simulink subsystem "DetailedBatteryModel"  (R2023b)
settings: Solver=VariableStepAuto  StartTime=0.0  StopTime=10.0  RelTol=1e-3
undefined symbols (not defined in the file): PlntBattBalSwtchThresh, PlntBattBleedRes, PlntBattCondArea, PlntBattNumCellPar, ThrmBatt1, ThrmBatt2, ThrmBatt3, ThrmBatt4
libraries: fl_lib x580, nesl_utility_internal x386, batteryecm_lib x96, simulink x96
(part 7 of 7)

== system DetailedBatteryModel/BatteryPack_16Modules/Cell_Module_2/s15 ==
  Compare To Constant4 : simulink/Logic and Bit Operations/Compare To Constant  relop=<=  const=0.001  OutDataTypeStr=boolean
  PS-Simulink Converter10 : nesl_utility_internal/PS-Simulink Converter  PhysicalDomain=network_engine_domain  SubClassName=ps_output  LeftPortType=input  RightPortType=output  PseudoPeriodic=off  Frequencies=[]  VectorFormat=1-D array  Unit=1  AffineConversion=off
  Stop Simulation4 : Stop
  p : PMIOPort  Side=Left
  wires:
  PS-Simulink Converter10/1 -> Compare To Constant4/1
  Compare To Constant4/1 -> Stop Simulation4/1
  connections:
  PS-Simulink Converter10/LConn1 -- p/RConn1

== system DetailedBatteryModel/BatteryPack_16Modules/Cell_Module_2/s16 ==
  Compare To Constant5 : simulink/Logic and Bit Operations/Compare To Constant  relop=<=  const=0.001  OutDataTypeStr=boolean
  PS-Simulink Converter11 : nesl_utility_internal/PS-Simulink Converter  PhysicalDomain=network_engine_domain  SubClassName=ps_output  LeftPortType=input  RightPortType=output  PseudoPeriodic=off  Frequencies=[]  VectorFormat=1-D array  Unit=1  AffineConversion=off
  Stop Simulation5 : Stop
  p : PMIOPort  Side=Left
  wires:
  PS-Simulink Converter11/1 -> Compare To Constant5/1
  Compare To Constant5/1 -> Stop Simulation5/1
  connections:
  PS-Simulink Converter11/LConn1 -- p/RConn1

== system DetailedBatteryModel/BatteryPack_16Modules/Cell_Module_2/s17 ==
  Compare To Constant1 : simulink/Logic and Bit Operations/Compare To Constant  relop=<=  const=0.001  OutDataTypeStr=boolean
  PS-Simulink Converter7 : nesl_utility_internal/PS-Simulink Converter  PhysicalDomain=network_engine_domain  SubClassName=ps_output  LeftPortType=input  RightPortType=output  PseudoPeriodic=off  Frequencies=[]  VectorFormat=1-D array  Unit=1  AffineConversion=off
  Stop Simulation1 : Stop
  p : PMIOPort  Side=Left
  wires:
  PS-Simulink Converter7/1 -> Compare To Constant1/1
  Compare To Constant1/1 -> Stop Simulation1/1
  connections:
  PS-Simulink Converter7/LConn1 -- p/RConn1

== system DetailedBatteryModel/BatteryPack_16Modules/Cell_Module_2/s18 ==
  Compare To Constant2 : simulink/Logic and Bit Operations/Compare To Constant  relop=<=  const=0.001  OutDataTypeStr=boolean
  PS-Simulink Converter8 : nesl_utility_internal/PS-Simulink Converter  PhysicalDomain=network_engine_domain  SubClassName=ps_output  LeftPortType=input  RightPortType=output  PseudoPeriodic=off  Frequencies=[]  VectorFormat=1-D array  Unit=1  AffineConversion=off
  Stop Simulation2 : Stop
  p : PMIOPort  Side=Left
  wires:
  Compare To Constant2/1 -> Stop Simulation2/1
  PS-Simulink Converter8/1 -> Compare To Constant2/1
  connections:
  PS-Simulink Converter8/LConn1 -- p/RConn1

== system DetailedBatteryModel/BatteryPack_16Modules/Cell_Module_2/s19 ==
  Compare To Constant3 : simulink/Logic and Bit Operations/Compare To Constant  relop=<=  const=0.001  OutDataTypeStr=boolean
  PS-Simulink Converter9 : nesl_utility_internal/PS-Simulink Converter  PhysicalDomain=network_engine_domain  SubClassName=ps_output  LeftPortType=input  RightPortType=output  PseudoPeriodic=off  Frequencies=[]  VectorFormat=1-D array  Unit=1  AffineConversion=off
  Stop Simulation3 : Stop
  p : PMIOPort  Side=Left
  wires:
  PS-Simulink Converter9/1 -> Compare To Constant3/1
  Compare To Constant3/1 -> Stop Simulation3/1
  connections:
  PS-Simulink Converter9/LConn1 -- p/RConn1

== system DetailedBatteryModel/BatteryPack_16Modules/Cell_Module_2/s2 ==
  Compare To Constant3 : simulink/Logic and Bit Operations/Compare To Constant  relop=<=  const=0.001  OutDataTypeStr=boolean
  PS-Simulink Converter9 : nesl_utility_internal/PS-Simulink Converter  PhysicalDomain=network_engine_domain  SubClassName=ps_output  LeftPortType=input  RightPortType=output  PseudoPeriodic=off  Frequencies=[]  VectorFormat=1-D array  Unit=1  AffineConversion=off
  Stop Simulation3 : Stop
  p : PMIOPort  Side=Left
  wires:
  PS-Simulink Converter9/1 -> Compare To Constant3/1
  Compare To Constant3/1 -> Stop Simulation3/1
  connections:
  PS-Simulink Converter9/LConn1 -- p/RConn1

== system DetailedBatteryModel/BatteryPack_16Modules/Cell_Module_2/s20 ==
  Compare To Constant4 : simulink/Logic and Bit Operations/Compare To Constant  relop=<=  const=0.001  OutDataTypeStr=boolean
  PS-Simulink Converter10 : nesl_utility_internal/PS-Simulink Converter  PhysicalDomain=network_engine_domain  SubClassName=ps_output  LeftPortType=input  RightPortType=output  PseudoPeriodic=off  Frequencies=[]  VectorFormat=1-D array  Unit=1  AffineConversion=off
  Stop Simulation4 : Stop
  p : PMIOPort  Side=Left
  wires:
  PS-Simulink Converter10/1 -> Compare To Constant4/1
  Compare To Constant4/1 -> Stop Simulation4/1
  connections:
  PS-Simulink Converter10/LConn1 -- p/RConn1

== system DetailedBatteryModel/BatteryPack_16Modules/Cell_Module_2/s21 ==
  Compare To Constant5 : simulink/Logic and Bit Operations/Compare To Constant  relop=<=  const=0.001  OutDataTypeStr=boolean
  PS-Simulink Converter11 : nesl_utility_internal/PS-Simulink Converter  PhysicalDomain=network_engine_domain  SubClassName=ps_output  LeftPortType=input  RightPortType=output  PseudoPeriodic=off  Frequencies=[]  VectorFormat=1-D array  Unit=1  AffineConversion=off
  Stop Simulation5 : Stop
  p : PMIOPort  Side=Left
  wires:
  PS-Simulink Converter11/1 -> Compare To Constant5/1
  Compare To Constant5/1 -> Stop Simulation5/1
  connections:
  PS-Simulink Converter11/LConn1 -- p/RConn1

== system DetailedBatteryModel/BatteryPack_16Modules/Cell_Module_2/s22 ==
  Compare To Constant5 : simulink/Logic and Bit Operations/Compare To Constant  relop=<=  const=0.001  OutDataTypeStr=boolean
  PS-Simulink Converter11 : nesl_utility_internal/PS-Simulink Converter  PhysicalDomain=network_engine_domain  SubClassName=ps_output  LeftPortType=input  RightPortType=output  PseudoPeriodic=off  Frequencies=[]  VectorFormat=1-D array  Unit=1  AffineConversion=off
  Stop Simulation5 : Stop
  p : PMIOPort  Side=Left
  wires:
  Compare To Constant5/1 -> Stop Simulation5/1
  PS-Simulink Converter11/1 -> Compare To Constant5/1
  connections:
  PS-Simulink Converter11/LConn1 -- p/RConn1

== system DetailedBatteryModel/BatteryPack_16Modules/Cell_Module_2/s3 ==
  Compare To Constant4 : simulink/Logic and Bit Operations/Compare To Constant  relop=<=  const=0.001  OutDataTypeStr=boolean
  PS-Simulink Converter10 : nesl_utility_internal/PS-Simulink Converter  PhysicalDomain=network_engine_domain  SubClassName=ps_output  LeftPortType=input  RightPortType=output  PseudoPeriodic=off  Frequencies=[]  VectorFormat=1-D array  Unit=1  AffineConversion=off
  Stop Simulation4 : Stop
  p : PMIOPort  Side=Left
  wires:
  PS-Simulink Converter10/1 -> Compare To Constant4/1
  Compare To Constant4/1 -> Stop Simulation4/1
  connections:
  PS-Simulink Converter10/LConn1 -- p/RConn1

== system DetailedBatteryModel/BatteryPack_16Modules/Cell_Module_2/s4 ==
  Compare To Constant5 : simulink/Logic and Bit Operations/Compare To Constant  relop=<=  const=0.001  OutDataTypeStr=boolean
  PS-Simulink Converter11 : nesl_utility_internal/PS-Simulink Converter  PhysicalDomain=network_engine_domain  SubClassName=ps_output  LeftPortType=input  RightPortType=output  PseudoPeriodic=off  Frequencies=[]  VectorFormat=1-D array  Unit=1  AffineConversion=off
  Stop Simulation5 : Stop
  p : PMIOPort  Side=Left
  wires:
  PS-Simulink Converter11/1 -> Compare To Constant5/1
  Compare To Constant5/1 -> Stop Simulation5/1
  connections:
  PS-Simulink Converter11/LConn1 -- p/RConn1

== system DetailedBatteryModel/BatteryPack_16Modules/Cell_Module_2/s5 ==
  Compare To Constant1 : simulink/Logic and Bit Operations/Compare To Constant  relop=<=  const=0.001  OutDataTypeStr=boolean
  PS-Simulink Converter7 : nesl_utility_internal/PS-Simulink Converter  PhysicalDomain=network_engine_domain  SubClassName=ps_output  LeftPortType=input  RightPortType=output  PseudoPeriodic=off  Frequencies=[]  VectorFormat=1-D array  Unit=1  AffineConversion=off
  Stop Simulation1 : Stop
  p : PMIOPort  Side=Left
  wires:
  PS-Simulink Converter7/1 -> Compare To Constant1/1
  Compare To Constant1/1 -> Stop Simulation1/1
  connections:
  PS-Simulink Converter7/LConn1 -- p/RConn1

== system DetailedBatteryModel/BatteryPack_16Modules/Cell_Module_2/s6 ==
  Compare To Constant2 : simulink/Logic and Bit Operations/Compare To Constant  relop=<=  const=0.001  OutDataTypeStr=boolean
  PS-Simulink Converter8 : nesl_utility_internal/PS-Simulink Converter  PhysicalDomain=network_engine_domain  SubClassName=ps_output  LeftPortType=input  RightPortType=output  PseudoPeriodic=off  Frequencies=[]  VectorFormat=1-D array  Unit=1  AffineConversion=off
  Stop Simulation2 : Stop
  p : PMIOPort  Side=Left
  wires:
  Compare To Constant2/1 -> Stop Simulation2/1
  PS-Simulink Converter8/1 -> Compare To Constant2/1
  connections:
  PS-Simulink Converter8/LConn1 -- p/RConn1

== system DetailedBatteryModel/BatteryPack_16Modules/Cell_Module_2/s7 ==
  Compare To Constant3 : simulink/Logic and Bit Operations/Compare To Constant  relop=<=  const=0.001  OutDataTypeStr=boolean
  PS-Simulink Converter9 : nesl_utility_internal/PS-Simulink Converter  PhysicalDomain=network_engine_domain  SubClassName=ps_output  LeftPortType=input  RightPortType=output  PseudoPeriodic=off  Frequencies=[]  VectorFormat=1-D array  Unit=1  AffineConversion=off
  Stop Simulation3 : Stop
  p : PMIOPort  Side=Left
  wires:
  PS-Simulink Converter9/1 -> Compare To Constant3/1
  Compare To Constant3/1 -> Stop Simulation3/1
  connections:
  PS-Simulink Converter9/LConn1 -- p/RConn1

== system DetailedBatteryModel/BatteryPack_16Modules/Cell_Module_2/s8 ==
  Compare To Constant4 : simulink/Logic and Bit Operations/Compare To Constant  relop=<=  const=0.001  OutDataTypeStr=boolean
  PS-Simulink Converter10 : nesl_utility_internal/PS-Simulink Converter  PhysicalDomain=network_engine_domain  SubClassName=ps_output  LeftPortType=input  RightPortType=output  PseudoPeriodic=off  Frequencies=[]  VectorFormat=1-D array  Unit=1  AffineConversion=off
  Stop Simulation4 : Stop
  p : PMIOPort  Side=Left
  wires:
  PS-Simulink Converter10/1 -> Compare To Constant4/1
  Compare To Constant4/1 -> Stop Simulation4/1
  connections:
  PS-Simulink Converter10/LConn1 -- p/RConn1

== system DetailedBatteryModel/BatteryPack_16Modules/Cell_Module_2/s9 ==
  Compare To Constant5 : simulink/Logic and Bit Operations/Compare To Constant  relop=<=  const=0.001  OutDataTypeStr=boolean
  PS-Simulink Converter11 : nesl_utility_internal/PS-Simulink Converter  PhysicalDomain=network_engine_domain  SubClassName=ps_output  LeftPortType=input  RightPortType=output  PseudoPeriodic=off  Frequencies=[]  VectorFormat=1-D array  Unit=1  AffineConversion=off
  Stop Simulation5 : Stop
  p : PMIOPort  Side=Left
  wires:
  PS-Simulink Converter11/1 -> Compare To Constant5/1
  Compare To Constant5/1 -> Stop Simulation5/1
  connections:
  PS-Simulink Converter11/LConn1 -- p/RConn1

== system DetailedBatteryModel/BatteryPack_16Modules/Cell_Module_3/Subsystem ==
  Compare To Constant : simulink/Logic and Bit Operations/Compare To Constant  relop=<=  const=0.001  OutDataTypeStr=boolean
  Data Type Conversion6 : DataTypeConversion  OutDataTypeStr=single  SaturateOnIntegerOverflow=off  RndMeth=Floor
  PS-Simulink Converter6 : nesl_utility_internal/PS-Simulink Converter  PhysicalDomain=network_engine_domain  SubClassName=ps_output  LeftPortType=input  RightPortType=output  PseudoPeriodic=off  Frequencies=[]  VectorFormat=1-D array  Unit=1  AffineConversion=off
  Stop Simulation : Stop
  P : PMIOPort  Side=Left
  soc : Outport
  wires:
  Data Type Conversion6/1 -> soc/1  "KnownSOC"
  PS-Simulink Converter6/1 -> Compare To Constant/1, Data Type Conversion6/1  "KnownSOC"
  Compare To Constant/1 -> Stop Simulation/1
  connections:
  P/RConn1 -- PS-Simulink Converter6/LConn1

== system DetailedBatteryModel/BatteryPack_16Modules/Cell_Module_3/s ==
  Compare To Constant1 : simulink/Logic and Bit Operations/Compare To Constant  relop=<=  const=0.001  OutDataTypeStr=boolean
  PS-Simulink Converter7 : nesl_utility_internal/PS-Simulink Converter  PhysicalDomain=network_engine_domain  SubClassName=ps_output  LeftPortType=input  RightPortType=output  PseudoPeriodic=off  Frequencies=[]  VectorFormat=1-D array  Unit=1  AffineConversion=off
  Stop Simulation1 : Stop
  p : PMIOPort  Side=Left
  wires:
  PS-Simulink Converter7/1 -> Compare To Constant1/1
  Compare To Constant1/1 -> Stop Simulation1/1
  connections:
  PS-Simulink Converter7/LConn1 -- p/RConn1

== system DetailedBatteryModel/BatteryPack_16Modules/Cell_Module_3/s1 ==
  Compare To Constant2 : simulink/Logic and Bit Operations/Compare To Constant  relop=<=  const=0.001  OutDataTypeStr=boolean
  PS-Simulink Converter8 : nesl_utility_internal/PS-Simulink Converter  PhysicalDomain=network_engine_domain  SubClassName=ps_output  LeftPortType=input  RightPortType=output  PseudoPeriodic=off  Frequencies=[]  VectorFormat=1-D array  Unit=1  AffineConversion=off
  Stop Simulation2 : Stop
  p : PMIOPort  Side=Left
  wires:
  Compare To Constant2/1 -> Stop Simulation2/1
  PS-Simulink Converter8/1 -> Compare To Constant2/1
  connections:
  PS-Simulink Converter8/LConn1 -- p/RConn1

== system DetailedBatteryModel/BatteryPack_16Modules/Cell_Module_3/s10 ==
  Compare To Constant5 : simulink/Logic and Bit Operations/Compare To Constant  relop=<=  const=0.001  OutDataTypeStr=boolean
  PS-Simulink Converter11 : nesl_utility_internal/PS-Simulink Converter  PhysicalDomain=network_engine_domain  SubClassName=ps_output  LeftPortType=input  RightPortType=output  PseudoPeriodic=off  Frequencies=[]  VectorFormat=1-D array  Unit=1  AffineConversion=off
  Stop Simulation5 : Stop
  p : PMIOPort  Side=Left
  wires:
  Compare To Constant5/1 -> Stop Simulation5/1
  PS-Simulink Converter11/1 -> Compare To Constant5/1
  connections:
  PS-Simulink Converter11/LConn1 -- p/RConn1

== system DetailedBatteryModel/BatteryPack_16Modules/Cell_Module_3/s11 ==
  Compare To Constant1 : simulink/Logic and Bit Operations/Compare To Constant  relop=<=  const=0.001  OutDataTypeStr=boolean
  PS-Simulink Converter7 : nesl_utility_internal/PS-Simulink Converter  PhysicalDomain=network_engine_domain  SubClassName=ps_output  LeftPortType=input  RightPortType=output  PseudoPeriodic=off  Frequencies=[]  VectorFormat=1-D array  Unit=1  AffineConversion=off
  Stop Simulation1 : Stop
  p : PMIOPort  Side=Left
  wires:
  PS-Simulink Converter7/1 -> Compare To Constant1/1
  Compare To Constant1/1 -> Stop Simulation1/1
  connections:
  PS-Simulink Converter7/LConn1 -- p/RConn1

== system DetailedBatteryModel/BatteryPack_16Modules/Cell_Module_3/s12 ==
  Compare To Constant2 : simulink/Logic and Bit Operations/Compare To Constant  relop=<=  const=0.001  OutDataTypeStr=boolean
  PS-Simulink Converter8 : nesl_utility_internal/PS-Simulink Converter  PhysicalDomain=network_engine_domain  SubClassName=ps_output  LeftPortType=input  RightPortType=output  PseudoPeriodic=off  Frequencies=[]  VectorFormat=1-D array  Unit=1  AffineConversion=off
  Stop Simulation2 : Stop
  p : PMIOPort  Side=Left
  wires:
  Compare To Constant2/1 -> Stop Simulation2/1
  PS-Simulink Converter8/1 -> Compare To Constant2/1
  connections:
  PS-Simulink Converter8/LConn1 -- p/RConn1

== system DetailedBatteryModel/BatteryPack_16Modules/Cell_Module_3/s13 ==
  Compare To Constant5 : simulink/Logic and Bit Operations/Compare To Constant  relop=<=  const=0.001  OutDataTypeStr=boolean
  PS-Simulink Converter11 : nesl_utility_internal/PS-Simulink Converter  PhysicalDomain=network_engine_domain  SubClassName=ps_output  LeftPortType=input  RightPortType=output  PseudoPeriodic=off  Frequencies=[]  VectorFormat=1-D array  Unit=1  AffineConversion=off
  Stop Simulation5 : Stop
  p : PMIOPort  Side=Left
  wires:
  Compare To Constant5/1 -> Stop Simulation5/1
  PS-Simulink Converter11/1 -> Compare To Constant5/1
  connections:
  PS-Simulink Converter11/LConn1 -- p/RConn1

== system DetailedBatteryModel/BatteryPack_16Modules/Cell_Module_3/s14 ==
  Compare To Constant3 : simulink/Logic and Bit Operations/Compare To Constant  relop=<=  const=0.001  OutDataTypeStr=boolean
  PS-Simulink Converter9 : nesl_utility_internal/PS-Simulink Converter  PhysicalDomain=network_engine_domain  SubClassName=ps_output  LeftPortType=input  RightPortType=output  PseudoPeriodic=off  Frequencies=[]  VectorFormat=1-D array  Unit=1  AffineConversion=off
  Stop Simulation3 : Stop
  p : PMIOPort  Side=Left
  wires:
  PS-Simulink Converter9/1 -> Compare To Constant3/1
  Compare To Constant3/1 -> Stop Simulation3/1
  connections:
  PS-Simulink Converter9/LConn1 -- p/RConn1

== system DetailedBatteryModel/BatteryPack_16Modules/Cell_Module_3/s15 ==
  Compare To Constant4 : simulink/Logic and Bit Operations/Compare To Constant  relop=<=  const=0.001  OutDataTypeStr=boolean
  PS-Simulink Converter10 : nesl_utility_internal/PS-Simulink Converter  PhysicalDomain=network_engine_domain  SubClassName=ps_output  LeftPortType=input  RightPortType=output  PseudoPeriodic=off  Frequencies=[]  VectorFormat=1-D array  Unit=1  AffineConversion=off
  Stop Simulation4 : Stop
  p : PMIOPort  Side=Left
  wires:
  PS-Simulink Converter10/1 -> Compare To Constant4/1
  Compare To Constant4/1 -> Stop Simulation4/1
  connections:
  PS-Simulink Converter10/LConn1 -- p/RConn1

== system DetailedBatteryModel/BatteryPack_16Modules/Cell_Module_3/s16 ==
  Compare To Constant5 : simulink/Logic and Bit Operations/Compare To Constant  relop=<=  const=0.001  OutDataTypeStr=boolean
  PS-Simulink Converter11 : nesl_utility_internal/PS-Simulink Converter  PhysicalDomain=network_engine_domain  SubClassName=ps_output  LeftPortType=input  RightPortType=output  PseudoPeriodic=off  Frequencies=[]  VectorFormat=1-D array  Unit=1  AffineConversion=off
  Stop Simulation5 : Stop
  p : PMIOPort  Side=Left
  wires:
  PS-Simulink Converter11/1 -> Compare To Constant5/1
  Compare To Constant5/1 -> Stop Simulation5/1
  connections:
  PS-Simulink Converter11/LConn1 -- p/RConn1

== system DetailedBatteryModel/BatteryPack_16Modules/Cell_Module_3/s17 ==
  Compare To Constant1 : simulink/Logic and Bit Operations/Compare To Constant  relop=<=  const=0.001  OutDataTypeStr=boolean
  PS-Simulink Converter7 : nesl_utility_internal/PS-Simulink Converter  PhysicalDomain=network_engine_domain  SubClassName=ps_output  LeftPortType=input  RightPortType=output  PseudoPeriodic=off  Frequencies=[]  VectorFormat=1-D array  Unit=1  AffineConversion=off
  Stop Simulation1 : Stop
  p : PMIOPort  Side=Left
  wires:
  PS-Simulink Converter7/1 -> Compare To Constant1/1
  Compare To Constant1/1 -> Stop Simulation1/1
  connections:
  PS-Simulink Converter7/LConn1 -- p/RConn1

== system DetailedBatteryModel/BatteryPack_16Modules/Cell_Module_3/s18 ==
  Compare To Constant2 : simulink/Logic and Bit Operations/Compare To Constant  relop=<=  const=0.001  OutDataTypeStr=boolean
  PS-Simulink Converter8 : nesl_utility_internal/PS-Simulink Converter  PhysicalDomain=network_engine_domain  SubClassName=ps_output  LeftPortType=input  RightPortType=output  PseudoPeriodic=off  Frequencies=[]  VectorFormat=1-D array  Unit=1  AffineConversion=off
  Stop Simulation2 : Stop
  p : PMIOPort  Side=Left
  wires:
  Compare To Constant2/1 -> Stop Simulation2/1
  PS-Simulink Converter8/1 -> Compare To Constant2/1
  connections:
  PS-Simulink Converter8/LConn1 -- p/RConn1

== system DetailedBatteryModel/BatteryPack_16Modules/Cell_Module_3/s19 ==
  Compare To Constant3 : simulink/Logic and Bit Operations/Compare To Constant  relop=<=  const=0.001  OutDataTypeStr=boolean
  PS-Simulink Converter9 : nesl_utility_internal/PS-Simulink Converter  PhysicalDomain=network_engine_domain  SubClassName=ps_output  LeftPortType=input  RightPortType=output  PseudoPeriodic=off  Frequencies=[]  VectorFormat=1-D array  Unit=1  AffineConversion=off
  Stop Simulation3 : Stop
  p : PMIOPort  Side=Left
  wires:
  PS-Simulink Converter9/1 -> Compare To Constant3/1
  Compare To Constant3/1 -> Stop Simulation3/1
  connections:
  PS-Simulink Converter9/LConn1 -- p/RConn1

== system DetailedBatteryModel/BatteryPack_16Modules/Cell_Module_3/s2 ==
  Compare To Constant3 : simulink/Logic and Bit Operations/Compare To Constant  relop=<=  const=0.001  OutDataTypeStr=boolean
  PS-Simulink Converter9 : nesl_utility_internal/PS-Simulink Converter  PhysicalDomain=network_engine_domain  SubClassName=ps_output  LeftPortType=input  RightPortType=output  PseudoPeriodic=off  Frequencies=[]  VectorFormat=1-D array  Unit=1  AffineConversion=off
  Stop Simulation3 : Stop
  p : PMIOPort  Side=Left
  wires:
  PS-Simulink Converter9/1 -> Compare To Constant3/1
  Compare To Constant3/1 -> Stop Simulation3/1
  connections:
  PS-Simulink Converter9/LConn1 -- p/RConn1

== system DetailedBatteryModel/BatteryPack_16Modules/Cell_Module_3/s20 ==
  Compare To Constant4 : simulink/Logic and Bit Operations/Compare To Constant  relop=<=  const=0.001  OutDataTypeStr=boolean
  PS-Simulink Converter10 : nesl_utility_internal/PS-Simulink Converter  PhysicalDomain=network_engine_domain  SubClassName=ps_output  LeftPortType=input  RightPortType=output  PseudoPeriodic=off  Frequencies=[]  VectorFormat=1-D array  Unit=1  AffineConversion=off
  Stop Simulation4 : Stop
  p : PMIOPort  Side=Left
  wires:
  PS-Simulink Converter10/1 -> Compare To Constant4/1
  Compare To Constant4/1 -> Stop Simulation4/1
  connections:
  PS-Simulink Converter10/LConn1 -- p/RConn1

== system DetailedBatteryModel/BatteryPack_16Modules/Cell_Module_3/s21 ==
  Compare To Constant5 : simulink/Logic and Bit Operations/Compare To Constant  relop=<=  const=0.001  OutDataTypeStr=boolean
  PS-Simulink Converter11 : nesl_utility_internal/PS-Simulink Converter  PhysicalDomain=network_engine_domain  SubClassName=ps_output  LeftPortType=input  RightPortType=output  PseudoPeriodic=off  Frequencies=[]  VectorFormat=1-D array  Unit=1  AffineConversion=off
  Stop Simulation5 : Stop
  p : PMIOPort  Side=Left
  wires:
  PS-Simulink Converter11/1 -> Compare To Constant5/1
  Compare To Constant5/1 -> Stop Simulation5/1
  connections:
  PS-Simulink Converter11/LConn1 -- p/RConn1

== system DetailedBatteryModel/BatteryPack_16Modules/Cell_Module_3/s22 ==
  Compare To Constant5 : simulink/Logic and Bit Operations/Compare To Constant  relop=<=  const=0.001  OutDataTypeStr=boolean
  PS-Simulink Converter11 : nesl_utility_internal/PS-Simulink Converter  PhysicalDomain=network_engine_domain  SubClassName=ps_output  LeftPortType=input  RightPortType=output  PseudoPeriodic=off  Frequencies=[]  VectorFormat=1-D array  Unit=1  AffineConversion=off
  Stop Simulation5 : Stop
  p : PMIOPort  Side=Left
  wires:
  Compare To Constant5/1 -> Stop Simulation5/1
  PS-Simulink Converter11/1 -> Compare To Constant5/1
  connections:
  PS-Simulink Converter11/LConn1 -- p/RConn1

== system DetailedBatteryModel/BatteryPack_16Modules/Cell_Module_3/s3 ==
  Compare To Constant4 : simulink/Logic and Bit Operations/Compare To Constant  relop=<=  const=0.001  OutDataTypeStr=boolean
  PS-Simulink Converter10 : nesl_utility_internal/PS-Simulink Converter  PhysicalDomain=network_engine_domain  SubClassName=ps_output  LeftPortType=input  RightPortType=output  PseudoPeriodic=off  Frequencies=[]  VectorFormat=1-D array  Unit=1  AffineConversion=off
  Stop Simulation4 : Stop
  p : PMIOPort  Side=Left
  wires:
  PS-Simulink Converter10/1 -> Compare To Constant4/1
  Compare To Constant4/1 -> Stop Simulation4/1
  connections:
  PS-Simulink Converter10/LConn1 -- p/RConn1

== system DetailedBatteryModel/BatteryPack_16Modules/Cell_Module_3/s4 ==
  Compare To Constant5 : simulink/Logic and Bit Operations/Compare To Constant  relop=<=  const=0.001  OutDataTypeStr=boolean
  PS-Simulink Converter11 : nesl_utility_internal/PS-Simulink Converter  PhysicalDomain=network_engine_domain  SubClassName=ps_output  LeftPortType=input  RightPortType=output  PseudoPeriodic=off  Frequencies=[]  VectorFormat=1-D array  Unit=1  AffineConversion=off
  Stop Simulation5 : Stop
  p : PMIOPort  Side=Left
  wires:
  PS-Simulink Converter11/1 -> Compare To Constant5/1
  Compare To Constant5/1 -> Stop Simulation5/1
  connections:
  PS-Simulink Converter11/LConn1 -- p/RConn1

== system DetailedBatteryModel/BatteryPack_16Modules/Cell_Module_3/s5 ==
  Compare To Constant1 : simulink/Logic and Bit Operations/Compare To Constant  relop=<=  const=0.001  OutDataTypeStr=boolean
  PS-Simulink Converter7 : nesl_utility_internal/PS-Simulink Converter  PhysicalDomain=network_engine_domain  SubClassName=ps_output  LeftPortType=input  RightPortType=output  PseudoPeriodic=off  Frequencies=[]  VectorFormat=1-D array  Unit=1  AffineConversion=off
  Stop Simulation1 : Stop
  p : PMIOPort  Side=Left
  wires:
  PS-Simulink Converter7/1 -> Compare To Constant1/1
  Compare To Constant1/1 -> Stop Simulation1/1
  connections:
  PS-Simulink Converter7/LConn1 -- p/RConn1

== system DetailedBatteryModel/BatteryPack_16Modules/Cell_Module_3/s6 ==
  Compare To Constant2 : simulink/Logic and Bit Operations/Compare To Constant  relop=<=  const=0.001  OutDataTypeStr=boolean
  PS-Simulink Converter8 : nesl_utility_internal/PS-Simulink Converter  PhysicalDomain=network_engine_domain  SubClassName=ps_output  LeftPortType=input  RightPortType=output  PseudoPeriodic=off  Frequencies=[]  VectorFormat=1-D array  Unit=1  AffineConversion=off
  Stop Simulation2 : Stop
  p : PMIOPort  Side=Left
  wires:
  Compare To Constant2/1 -> Stop Simulation2/1
  PS-Simulink Converter8/1 -> Compare To Constant2/1
  connections:
  PS-Simulink Converter8/LConn1 -- p/RConn1

== system DetailedBatteryModel/BatteryPack_16Modules/Cell_Module_3/s7 ==
  Compare To Constant3 : simulink/Logic and Bit Operations/Compare To Constant  relop=<=  const=0.001  OutDataTypeStr=boolean
  PS-Simulink Converter9 : nesl_utility_internal/PS-Simulink Converter  PhysicalDomain=network_engine_domain  SubClassName=ps_output  LeftPortType=input  RightPortType=output  PseudoPeriodic=off  Frequencies=[]  VectorFormat=1-D array  Unit=1  AffineConversion=off
  Stop Simulation3 : Stop
  p : PMIOPort  Side=Left
  wires:
  PS-Simulink Converter9/1 -> Compare To Constant3/1
  Compare To Constant3/1 -> Stop Simulation3/1
  connections:
  PS-Simulink Converter9/LConn1 -- p/RConn1

== system DetailedBatteryModel/BatteryPack_16Modules/Cell_Module_3/s8 ==
  Compare To Constant4 : simulink/Logic and Bit Operations/Compare To Constant  relop=<=  const=0.001  OutDataTypeStr=boolean
  PS-Simulink Converter10 : nesl_utility_internal/PS-Simulink Converter  PhysicalDomain=network_engine_domain  SubClassName=ps_output  LeftPortType=input  RightPortType=output  PseudoPeriodic=off  Frequencies=[]  VectorFormat=1-D array  Unit=1  AffineConversion=off
  Stop Simulation4 : Stop
  p : PMIOPort  Side=Left
  wires:
  PS-Simulink Converter10/1 -> Compare To Constant4/1
  Compare To Constant4/1 -> Stop Simulation4/1
  connections:
  PS-Simulink Converter10/LConn1 -- p/RConn1

== system DetailedBatteryModel/BatteryPack_16Modules/Cell_Module_3/s9 ==
  Compare To Constant5 : simulink/Logic and Bit Operations/Compare To Constant  relop=<=  const=0.001  OutDataTypeStr=boolean
  PS-Simulink Converter11 : nesl_utility_internal/PS-Simulink Converter  PhysicalDomain=network_engine_domain  SubClassName=ps_output  LeftPortType=input  RightPortType=output  PseudoPeriodic=off  Frequencies=[]  VectorFormat=1-D array  Unit=1  AffineConversion=off
  Stop Simulation5 : Stop
  p : PMIOPort  Side=Left
  wires:
  PS-Simulink Converter11/1 -> Compare To Constant5/1
  Compare To Constant5/1 -> Stop Simulation5/1
  connections:
  PS-Simulink Converter11/LConn1 -- p/RConn1

== system DetailedBatteryModel/BatteryPack_16Modules/Cell_Module_4/Subsystem ==
  Compare To Constant : simulink/Logic and Bit Operations/Compare To Constant  relop=<=  const=0.001  OutDataTypeStr=boolean
  Data Type Conversion6 : DataTypeConversion  OutDataTypeStr=single  SaturateOnIntegerOverflow=off  RndMeth=Floor
  PS-Simulink Converter6 : nesl_utility_internal/PS-Simulink Converter  PhysicalDomain=network_engine_domain  SubClassName=ps_output  LeftPortType=input  RightPortType=output  PseudoPeriodic=off  Frequencies=[]  VectorFormat=1-D array  Unit=1  AffineConversion=off
  Stop Simulation : Stop
  P : PMIOPort  Side=Left
  soc : Outport
  wires:
  Data Type Conversion6/1 -> soc/1  "KnownSOC"
  PS-Simulink Converter6/1 -> Compare To Constant/1, Data Type Conversion6/1  "KnownSOC"
  Compare To Constant/1 -> Stop Simulation/1
  connections:
  P/RConn1 -- PS-Simulink Converter6/LConn1

== system DetailedBatteryModel/BatteryPack_16Modules/Cell_Module_4/s ==
  Compare To Constant1 : simulink/Logic and Bit Operations/Compare To Constant  relop=<=  const=0.001  OutDataTypeStr=boolean
  PS-Simulink Converter7 : nesl_utility_internal/PS-Simulink Converter  PhysicalDomain=network_engine_domain  SubClassName=ps_output  LeftPortType=input  RightPortType=output  PseudoPeriodic=off  Frequencies=[]  VectorFormat=1-D array  Unit=1  AffineConversion=off
  Stop Simulation1 : Stop
  p : PMIOPort  Side=Left
  wires:
  PS-Simulink Converter7/1 -> Compare To Constant1/1
  Compare To Constant1/1 -> Stop Simulation1/1
  connections:
  PS-Simulink Converter7/LConn1 -- p/RConn1

== system DetailedBatteryModel/BatteryPack_16Modules/Cell_Module_4/s1 ==
  Compare To Constant2 : simulink/Logic and Bit Operations/Compare To Constant  relop=<=  const=0.001  OutDataTypeStr=boolean
  PS-Simulink Converter8 : nesl_utility_internal/PS-Simulink Converter  PhysicalDomain=network_engine_domain  SubClassName=ps_output  LeftPortType=input  RightPortType=output  PseudoPeriodic=off  Frequencies=[]  VectorFormat=1-D array  Unit=1  AffineConversion=off
  Stop Simulation2 : Stop
  p : PMIOPort  Side=Left
  wires:
  Compare To Constant2/1 -> Stop Simulation2/1
  PS-Simulink Converter8/1 -> Compare To Constant2/1
  connections:
  PS-Simulink Converter8/LConn1 -- p/RConn1

== system DetailedBatteryModel/BatteryPack_16Modules/Cell_Module_4/s10 ==
  Compare To Constant5 : simulink/Logic and Bit Operations/Compare To Constant  relop=<=  const=0.001  OutDataTypeStr=boolean
  PS-Simulink Converter11 : nesl_utility_internal/PS-Simulink Converter  PhysicalDomain=network_engine_domain  SubClassName=ps_output  LeftPortType=input  RightPortType=output  PseudoPeriodic=off  Frequencies=[]  VectorFormat=1-D array  Unit=1  AffineConversion=off
  Stop Simulation5 : Stop
  p : PMIOPort  Side=Left
  wires:
  Compare To Constant5/1 -> Stop Simulation5/1
  PS-Simulink Converter11/1 -> Compare To Constant5/1
  connections:
  PS-Simulink Converter11/LConn1 -- p/RConn1

== system DetailedBatteryModel/BatteryPack_16Modules/Cell_Module_4/s11 ==
  Compare To Constant1 : simulink/Logic and Bit Operations/Compare To Constant  relop=<=  const=0.001  OutDataTypeStr=boolean
  PS-Simulink Converter7 : nesl_utility_internal/PS-Simulink Converter  PhysicalDomain=network_engine_domain  SubClassName=ps_output  LeftPortType=input  RightPortType=output  PseudoPeriodic=off  Frequencies=[]  VectorFormat=1-D array  Unit=1  AffineConversion=off
  Stop Simulation1 : Stop
  p : PMIOPort  Side=Left
  wires:
  PS-Simulink Converter7/1 -> Compare To Constant1/1
  Compare To Constant1/1 -> Stop Simulation1/1
  connections:
  PS-Simulink Converter7/LConn1 -- p/RConn1

== system DetailedBatteryModel/BatteryPack_16Modules/Cell_Module_4/s12 ==
  Compare To Constant2 : simulink/Logic and Bit Operations/Compare To Constant  relop=<=  const=0.001  OutDataTypeStr=boolean
  PS-Simulink Converter8 : nesl_utility_internal/PS-Simulink Converter  PhysicalDomain=network_engine_domain  SubClassName=ps_output  LeftPortType=input  RightPortType=output  PseudoPeriodic=off  Frequencies=[]  VectorFormat=1-D array  Unit=1  AffineConversion=off
  Stop Simulation2 : Stop
  p : PMIOPort  Side=Left
  wires:
  Compare To Constant2/1 -> Stop Simulation2/1
  PS-Simulink Converter8/1 -> Compare To Constant2/1
  connections:
  PS-Simulink Converter8/LConn1 -- p/RConn1

== system DetailedBatteryModel/BatteryPack_16Modules/Cell_Module_4/s13 ==
  Compare To Constant5 : simulink/Logic and Bit Operations/Compare To Constant  relop=<=  const=0.001  OutDataTypeStr=boolean
  PS-Simulink Converter11 : nesl_utility_internal/PS-Simulink Converter  PhysicalDomain=network_engine_domain  SubClassName=ps_output  LeftPortType=input  RightPortType=output  PseudoPeriodic=off  Frequencies=[]  VectorFormat=1-D array  Unit=1  AffineConversion=off
  Stop Simulation5 : Stop
  p : PMIOPort  Side=Left
  wires:
  Compare To Constant5/1 -> Stop Simulation5/1
  PS-Simulink Converter11/1 -> Compare To Constant5/1
  connections:
  PS-Simulink Converter11/LConn1 -- p/RConn1

== system DetailedBatteryModel/BatteryPack_16Modules/Cell_Module_4/s14 ==
  Compare To Constant3 : simulink/Logic and Bit Operations/Compare To Constant  relop=<=  const=0.001  OutDataTypeStr=boolean
  PS-Simulink Converter9 : nesl_utility_internal/PS-Simulink Converter  PhysicalDomain=network_engine_domain  SubClassName=ps_output  LeftPortType=input  RightPortType=output  PseudoPeriodic=off  Frequencies=[]  VectorFormat=1-D array  Unit=1  AffineConversion=off
  Stop Simulation3 : Stop
  p : PMIOPort  Side=Left
  wires:
  PS-Simulink Converter9/1 -> Compare To Constant3/1
  Compare To Constant3/1 -> Stop Simulation3/1
  connections:
  PS-Simulink Converter9/LConn1 -- p/RConn1

== system DetailedBatteryModel/BatteryPack_16Modules/Cell_Module_4/s15 ==
  Compare To Constant4 : simulink/Logic and Bit Operations/Compare To Constant  relop=<=  const=0.001  OutDataTypeStr=boolean
  PS-Simulink Converter10 : nesl_utility_internal/PS-Simulink Converter  PhysicalDomain=network_engine_domain  SubClassName=ps_output  LeftPortType=input  RightPortType=output  PseudoPeriodic=off  Frequencies=[]  VectorFormat=1-D array  Unit=1  AffineConversion=off
  Stop Simulation4 : Stop
  p : PMIOPort  Side=Left
  wires:
  PS-Simulink Converter10/1 -> Compare To Constant4/1
  Compare To Constant4/1 -> Stop Simulation4/1
  connections:
  PS-Simulink Converter10/LConn1 -- p/RConn1

== system DetailedBatteryModel/BatteryPack_16Modules/Cell_Module_4/s16 ==
  Compare To Constant5 : simulink/Logic and Bit Operations/Compare To Constant  relop=<=  const=0.001  OutDataTypeStr=boolean
  PS-Simulink Converter11 : nesl_utility_internal/PS-Simulink Converter  PhysicalDomain=network_engine_domain  SubClassName=ps_output  LeftPortType=input  RightPortType=output  PseudoPeriodic=off  Frequencies=[]  VectorFormat=1-D array  Unit=1  AffineConversion=off
  Stop Simulation5 : Stop
  p : PMIOPort  Side=Left
  wires:
  PS-Simulink Converter11/1 -> Compare To Constant5/1
  Compare To Constant5/1 -> Stop Simulation5/1
  connections:
  PS-Simulink Converter11/LConn1 -- p/RConn1

== system DetailedBatteryModel/BatteryPack_16Modules/Cell_Module_4/s17 ==
  Compare To Constant1 : simulink/Logic and Bit Operations/Compare To Constant  relop=<=  const=0.001  OutDataTypeStr=boolean
  PS-Simulink Converter7 : nesl_utility_internal/PS-Simulink Converter  PhysicalDomain=network_engine_domain  SubClassName=ps_output  LeftPortType=input  RightPortType=output  PseudoPeriodic=off  Frequencies=[]  VectorFormat=1-D array  Unit=1  AffineConversion=off
  Stop Simulation1 : Stop
  p : PMIOPort  Side=Left
  wires:
  PS-Simulink Converter7/1 -> Compare To Constant1/1
  Compare To Constant1/1 -> Stop Simulation1/1
  connections:
  PS-Simulink Converter7/LConn1 -- p/RConn1

== system DetailedBatteryModel/BatteryPack_16Modules/Cell_Module_4/s18 ==
  Compare To Constant2 : simulink/Logic and Bit Operations/Compare To Constant  relop=<=  const=0.001  OutDataTypeStr=boolean
  PS-Simulink Converter8 : nesl_utility_internal/PS-Simulink Converter  PhysicalDomain=network_engine_domain  SubClassName=ps_output  LeftPortType=input  RightPortType=output  PseudoPeriodic=off  Frequencies=[]  VectorFormat=1-D array  Unit=1  AffineConversion=off
  Stop Simulation2 : Stop
  p : PMIOPort  Side=Left
  wires:
  Compare To Constant2/1 -> Stop Simulation2/1
  PS-Simulink Converter8/1 -> Compare To Constant2/1
  connections:
  PS-Simulink Converter8/LConn1 -- p/RConn1

== system DetailedBatteryModel/BatteryPack_16Modules/Cell_Module_4/s19 ==
  Compare To Constant3 : simulink/Logic and Bit Operations/Compare To Constant  relop=<=  const=0.001  OutDataTypeStr=boolean
  PS-Simulink Converter9 : nesl_utility_internal/PS-Simulink Converter  PhysicalDomain=network_engine_domain  SubClassName=ps_output  LeftPortType=input  RightPortType=output  PseudoPeriodic=off  Frequencies=[]  VectorFormat=1-D array  Unit=1  AffineConversion=off
  Stop Simulation3 : Stop
  p : PMIOPort  Side=Left
  wires:
  PS-Simulink Converter9/1 -> Compare To Constant3/1
  Compare To Constant3/1 -> Stop Simulation3/1
  connections:
  PS-Simulink Converter9/LConn1 -- p/RConn1

== system DetailedBatteryModel/BatteryPack_16Modules/Cell_Module_4/s2 ==
  Compare To Constant3 : simulink/Logic and Bit Operations/Compare To Constant  relop=<=  const=0.001  OutDataTypeStr=boolean
  PS-Simulink Converter9 : nesl_utility_internal/PS-Simulink Converter  PhysicalDomain=network_engine_domain  SubClassName=ps_output  LeftPortType=input  RightPortType=output  PseudoPeriodic=off  Frequencies=[]  VectorFormat=1-D array  Unit=1  AffineConversion=off
  Stop Simulation3 : Stop
  p : PMIOPort  Side=Left
  wires:
  PS-Simulink Converter9/1 -> Compare To Constant3/1
  Compare To Constant3/1 -> Stop Simulation3/1
  connections:
  PS-Simulink Converter9/LConn1 -- p/RConn1

== system DetailedBatteryModel/BatteryPack_16Modules/Cell_Module_4/s20 ==
  Compare To Constant4 : simulink/Logic and Bit Operations/Compare To Constant  relop=<=  const=0.001  OutDataTypeStr=boolean
  PS-Simulink Converter10 : nesl_utility_internal/PS-Simulink Converter  PhysicalDomain=network_engine_domain  SubClassName=ps_output  LeftPortType=input  RightPortType=output  PseudoPeriodic=off  Frequencies=[]  VectorFormat=1-D array  Unit=1  AffineConversion=off
  Stop Simulation4 : Stop
  p : PMIOPort  Side=Left
  wires:
  PS-Simulink Converter10/1 -> Compare To Constant4/1
  Compare To Constant4/1 -> Stop Simulation4/1
  connections:
  PS-Simulink Converter10/LConn1 -- p/RConn1

== system DetailedBatteryModel/BatteryPack_16Modules/Cell_Module_4/s21 ==
  Compare To Constant5 : simulink/Logic and Bit Operations/Compare To Constant  relop=<=  const=0.001  OutDataTypeStr=boolean
  PS-Simulink Converter11 : nesl_utility_internal/PS-Simulink Converter  PhysicalDomain=network_engine_domain  SubClassName=ps_output  LeftPortType=input  RightPortType=output  PseudoPeriodic=off  Frequencies=[]  VectorFormat=1-D array  Unit=1  AffineConversion=off
  Stop Simulation5 : Stop
  p : PMIOPort  Side=Left
  wires:
  PS-Simulink Converter11/1 -> Compare To Constant5/1
  Compare To Constant5/1 -> Stop Simulation5/1
  connections:
  PS-Simulink Converter11/LConn1 -- p/RConn1

== system DetailedBatteryModel/BatteryPack_16Modules/Cell_Module_4/s22 ==
  Compare To Constant5 : simulink/Logic and Bit Operations/Compare To Constant  relop=<=  const=0.001  OutDataTypeStr=boolean
  PS-Simulink Converter11 : nesl_utility_internal/PS-Simulink Converter  PhysicalDomain=network_engine_domain  SubClassName=ps_output  LeftPortType=input  RightPortType=output  PseudoPeriodic=off  Frequencies=[]  VectorFormat=1-D array  Unit=1  AffineConversion=off
  Stop Simulation5 : Stop
  p : PMIOPort  Side=Left
  wires:
  Compare To Constant5/1 -> Stop Simulation5/1
  PS-Simulink Converter11/1 -> Compare To Constant5/1
  connections:
  PS-Simulink Converter11/LConn1 -- p/RConn1

== system DetailedBatteryModel/BatteryPack_16Modules/Cell_Module_4/s3 ==
  Compare To Constant4 : simulink/Logic and Bit Operations/Compare To Constant  relop=<=  const=0.001  OutDataTypeStr=boolean
  PS-Simulink Converter10 : nesl_utility_internal/PS-Simulink Converter  PhysicalDomain=network_engine_domain  SubClassName=ps_output  LeftPortType=input  RightPortType=output  PseudoPeriodic=off  Frequencies=[]  VectorFormat=1-D array  Unit=1  AffineConversion=off
  Stop Simulation4 : Stop
  p : PMIOPort  Side=Left
  wires:
  PS-Simulink Converter10/1 -> Compare To Constant4/1
  Compare To Constant4/1 -> Stop Simulation4/1
  connections:
  PS-Simulink Converter10/LConn1 -- p/RConn1

== system DetailedBatteryModel/BatteryPack_16Modules/Cell_Module_4/s4 ==
  Compare To Constant5 : simulink/Logic and Bit Operations/Compare To Constant  relop=<=  const=0.001  OutDataTypeStr=boolean
  PS-Simulink Converter11 : nesl_utility_internal/PS-Simulink Converter  PhysicalDomain=network_engine_domain  SubClassName=ps_output  LeftPortType=input  RightPortType=output  PseudoPeriodic=off  Frequencies=[]  VectorFormat=1-D array  Unit=1  AffineConversion=off
  Stop Simulation5 : Stop
  p : PMIOPort  Side=Left
  wires:
  PS-Simulink Converter11/1 -> Compare To Constant5/1
  Compare To Constant5/1 -> Stop Simulation5/1
  connections:
  PS-Simulink Converter11/LConn1 -- p/RConn1

== system DetailedBatteryModel/BatteryPack_16Modules/Cell_Module_4/s5 ==
  Compare To Constant1 : simulink/Logic and Bit Operations/Compare To Constant  relop=<=  const=0.001  OutDataTypeStr=boolean
  PS-Simulink Converter7 : nesl_utility_internal/PS-Simulink Converter  PhysicalDomain=network_engine_domain  SubClassName=ps_output  LeftPortType=input  RightPortType=output  PseudoPeriodic=off  Frequencies=[]  VectorFormat=1-D array  Unit=1  AffineConversion=off
  Stop Simulation1 : Stop
  p : PMIOPort  Side=Left
  wires:
  PS-Simulink Converter7/1 -> Compare To Constant1/1
  Compare To Constant1/1 -> Stop Simulation1/1
  connections:
  PS-Simulink Converter7/LConn1 -- p/RConn1

== system DetailedBatteryModel/BatteryPack_16Modules/Cell_Module_4/s6 ==
  Compare To Constant2 : simulink/Logic and Bit Operations/Compare To Constant  relop=<=  const=0.001  OutDataTypeStr=boolean
  PS-Simulink Converter8 : nesl_utility_internal/PS-Simulink Converter  PhysicalDomain=network_engine_domain  SubClassName=ps_output  LeftPortType=input  RightPortType=output  PseudoPeriodic=off  Frequencies=[]  VectorFormat=1-D array  Unit=1  AffineConversion=off
  Stop Simulation2 : Stop
  p : PMIOPort  Side=Left
  wires:
  Compare To Constant2/1 -> Stop Simulation2/1
  PS-Simulink Converter8/1 -> Compare To Constant2/1
  connections:
  PS-Simulink Converter8/LConn1 -- p/RConn1

== system DetailedBatteryModel/BatteryPack_16Modules/Cell_Module_4/s7 ==
  Compare To Constant3 : simulink/Logic and Bit Operations/Compare To Constant  relop=<=  const=0.001  OutDataTypeStr=boolean
  PS-Simulink Converter9 : nesl_utility_internal/PS-Simulink Converter  PhysicalDomain=network_engine_domain  SubClassName=ps_output  LeftPortType=input  RightPortType=output  PseudoPeriodic=off  Frequencies=[]  VectorFormat=1-D array  Unit=1  AffineConversion=off
  Stop Simulation3 : Stop
  p : PMIOPort  Side=Left
  wires:
  PS-Simulink Converter9/1 -> Compare To Constant3/1
  Compare To Constant3/1 -> Stop Simulation3/1
  connections:
  PS-Simulink Converter9/LConn1 -- p/RConn1

== system DetailedBatteryModel/BatteryPack_16Modules/Cell_Module_4/s8 ==
  Compare To Constant4 : simulink/Logic and Bit Operations/Compare To Constant  relop=<=  const=0.001  OutDataTypeStr=boolean
  PS-Simulink Converter10 : nesl_utility_internal/PS-Simulink Converter  PhysicalDomain=network_engine_domain  SubClassName=ps_output  LeftPortType=input  RightPortType=output  PseudoPeriodic=off  Frequencies=[]  VectorFormat=1-D array  Unit=1  AffineConversion=off
  Stop Simulation4 : Stop
  p : PMIOPort  Side=Left
  wires:
  PS-Simulink Converter10/1 -> Compare To Constant4/1
  Compare To Constant4/1 -> Stop Simulation4/1
  connections:
  PS-Simulink Converter10/LConn1 -- p/RConn1

== system DetailedBatteryModel/BatteryPack_16Modules/Cell_Module_4/s9 ==
  Compare To Constant5 : simulink/Logic and Bit Operations/Compare To Constant  relop=<=  const=0.001  OutDataTypeStr=boolean
  PS-Simulink Converter11 : nesl_utility_internal/PS-Simulink Converter  PhysicalDomain=network_engine_domain  SubClassName=ps_output  LeftPortType=input  RightPortType=output  PseudoPeriodic=off  Frequencies=[]  VectorFormat=1-D array  Unit=1  AffineConversion=off
  Stop Simulation5 : Stop
  p : PMIOPort  Side=Left
  wires:
  PS-Simulink Converter11/1 -> Compare To Constant5/1
  Compare To Constant5/1 -> Stop Simulation5/1
  connections:
  PS-Simulink Converter11/LConn1 -- p/RConn1
